simulink model "nav2"  (R2020a)
settings: Solver=FixedStepAuto  StartTime=0.0  StopTime=inf  RelTol=1e-3
model workspace (MAT data in the model file):
  SL_ROS_VariableLengthArrays_MaxSizes.CommonInfo.ArrayTruncateAction = 'EmitWarning'
  SL_ROS_VariableLengthArrays_MaxSizes.MsgTypeMap = containers.Map
  SL_ROS_VariableLengthArrays_MaxSizes.MsgTypeMap.serialization.keys = {'nav_msgs/OccupancyGrid'}
  SL_ROS_VariableLengthArrays_MaxSizes.MsgTypeMap.serialization.values{1}.PropertyName = 'Data'
  SL_ROS_VariableLengthArrays_MaxSizes.MsgTypeMap.serialization.values{1}.DataType = 'int8'
  SL_ROS_VariableLengthArrays_MaxSizes.MsgTypeMap.serialization.values{1}.MaxLength = 1000000
  SL_ROS_VariableLengthArrays_MaxSizes.MsgTypeMap.serialization.uniformity = 0
  SL_ROS_VariableLengthArrays_MaxSizes.MsgTypeMap.serialization.keyType = 'char'
  SL_ROS_VariableLengthArrays_MaxSizes.MsgTypeMap.serialization.valueType = 'any'
values from neighbouring files (symbols this model uses):
  chargingStn = [setInitialPose(1,1), setInitialPose(1,2)]    [startup.m]
  L2RTransform = [cos(L2Rtheta), -sin(L2Rtheta), L2Rx ... (first row only)    [startup.m]
  LIVE_MODE = 0    [startup.m]
  loadingStn = [15, 15]    [startup.m]
  map = binaryOccupancyMap(logicalMap, 1/0.05)    [exampleHelperVisualizeExecuteRobots.m]
  unloadingStn = [15, 15]    [startup.m]
  W2LOTransform = W2ORTransform/(L2RTransform)    [startup.m]
  wheelBase = 0.4464    [startup.m]
  wheelRadius = 0.1715/2    (= 0.08575)    [startup.m]
undefined symbols (not defined in the file or in its folder): Angular, gray, Linear
libraries: robotlib x7, robotalgslib x2, vrlib x1
settings Model: EnablePacing=on  Creator=john  LastModifiedBy=jhtran
settings OptimizationCC: EnhancedBackFolding=on  PassReuseOutputArgsAs=Individual arguments  ZeroExternalMemoryAtStartup=off  ZeroInternalMemoryAtStartup=off  MaxStackSize=64  OptimizeBlockOrder=speed  DifferentSizesBufferReuse=on  OptimizationCustomize=off  EfficientTunableParamExpr=on
settings DebuggingCC: ParameterTunabilityLossMsg=error
settings HardwareCC: ProdBitPerPointer=32  ProdBitPerSizeT=32  ProdBitPerPtrDiffT=32  ProdLargestAtomicFloat=None  ProdIntDivRoundTo=Undefined  ProdEndianess=Unspecified  ProdWordSize=32  ProdHWDeviceType=Generic->Unspecified (assume 32-bit Generic)  UseEmbeddedCoderFeatures=off
settings RTWCC: SystemTargetFile=ert.tlc  HardwareBoard=Robot Operating System (ROS)  TemplateMakefile=ert_default_tmf  Toolchain=Catkin  TargetLang=C++
settings CodeAppCC: ForceParamTrailComments=on  IgnoreCustomStorageClasses=off  OperatorAnnotations=on  SimulinkDataObjDesc=on  SFDataObjDesc=on  InsertBlockDesc=on
settings ERTTargetCC: SupportNonInlinedSFcns=on

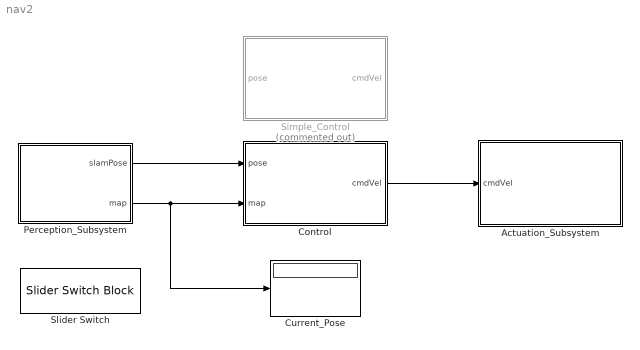
== system nav2 ==
  Actuation_Subsystem : Subsystem
  Control : Subsystem
  Current_Pose : Display
  Perception_Subsystem : Subsystem
  Simple_Control : Subsystem  Commented=on
  Slider Switch : SliderSwitchBlock
      settings: Values={{'Off', 'On'}, [0 1]}
  wires:
  Perception_Subsystem/1(slamPose) -> Control/1(pose)
  Control/1(cmdVel) -> Actuation_Subsystem/1(cmdVel)
  Perception_Subsystem/2(map) -> Current_Pose/1, Control/2(map)

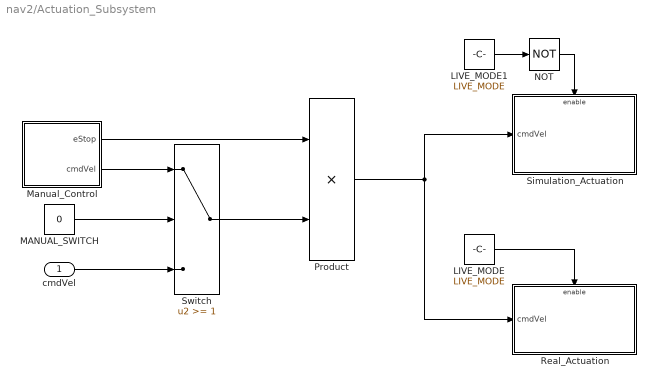
== system nav2/Actuation_Subsystem ==
  cmdVel : Inport
  LIVE_MODE : Constant  Value=LIVE_MODE
  LIVE_MODE1 : Constant  Value=LIVE_MODE
  MANUAL_SWITCH : Constant  Value=0
  Manual_Control : Subsystem
  NOT : Logic  Operator=NOT  IconShape=distinctive  AllPortsSameDT=off  OutDataTypeStr=boolean
  Product : Product
  Real_Actuation : Subsystem
  Simulation_Actuation : Subsystem
  Switch : Switch  Threshold=1
  wires:
  cmdVel/1 -> Switch/3
  Manual_Control/2(cmdVel) -> Switch/1
  MANUAL_SWITCH/1 -> Switch/2
  LIVE_MODE/1 -> Real_Actuation/Enable
  NOT/1 -> Simulation_Actuation/Enable
  LIVE_MODE1/1 -> NOT/1
  Switch/1 -> Product/2
  Product/1 -> Real_Actuation/1(cmdVel), Simulation_Actuation/1(cmdVel)
  Manual_Control/1(eStop) -> Product/1

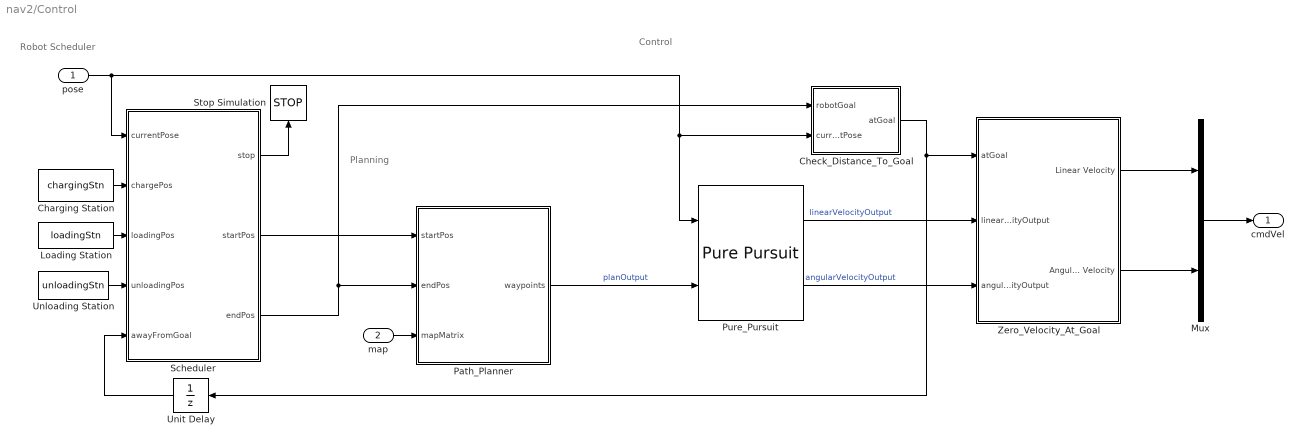
== system nav2/Control ==
  note: Control
  note: Robot Scheduler
  note: Planning
  pose : Inport
  map : Inport  Port=2
  "Charging Station " : Constant  Value=chargingStn  SampleTime=1
  Check_Distance_To_Goal : Subsystem
  Loading Station : Constant  Value=loadingStn
  Mux : Mux  Inputs=2
  Path_Planner : MATLAB Function  TreatAsAtomicUnit=on
  Pure_Pursuit : robotalgslib/Pure Pursuit  DesiredLinearVelocity=1  MaxAngularVelocity=0.5  LookaheadDistance=1  TargetDirPort=off  SimulateUsing=Code generation
  Scheduler : Stateflow chart  TreatAsAtomicUnit=on
  Stop Simulation : Stop
  Unit Delay : UnitDelay  SampleTime=-1  HasFrameUpgradeWarning=on
  Unloading Station : Constant  Value=unloadingStn  SampleTime=1
  Zero_Velocity_At_Goal : Subsystem
  cmdVel : Outport
  wires:
  Check_Distance_To_Goal/1(atGoal) -> Unit Delay/1, Zero_Velocity_At_Goal/1(atGoal)
  "Charging Station "/1 -> Scheduler/2(chargePos)
  Scheduler/2(startPos) -> Path_Planner/1(startPos)
  Unit Delay/1 -> Scheduler/5(awayFromGoal)
  Scheduler/3(endPos) -> Path_Planner/2(endPos), Check_Distance_To_Goal/1(robotGoal)
  Loading Station/1 -> Scheduler/3(loadingPos)
  Pure_Pursuit/2 -> Zero_Velocity_At_Goal/3(angularVelocityOutput)  "angularVelocityOutput"
  pose/1 -> Check_Distance_To_Goal/2(currentPose), Pure_Pursuit/1, Scheduler/1(currentPose)
  Unloading Station/1 -> Scheduler/4(unloadingPos)
  Scheduler/1(stop) -> Stop Simulation/1
  Path_Planner/1(waypoints) -> Pure_Pursuit/2  "planOutput"
  Pure_Pursuit/1 -> Zero_Velocity_At_Goal/2(linearVelocityOutput)  "linearVelocityOutput"
  Zero_Velocity_At_Goal/2(Angular Velocity) -> Mux/2
  Zero_Velocity_At_Goal/1(Linear Velocity) -> Mux/1
  Mux/1 -> cmdVel/1
  map/1 -> Path_Planner/3(mapMatrix)

== system nav2/Perception_Subsystem ==
  SLAM_Subsystem : Subsystem
  slamPose : Outport
  map : Outport  Port=2
  wires:
  SLAM_Subsystem/1(slamPose) -> slamPose/1
  SLAM_Subsystem/2(map) -> map/1

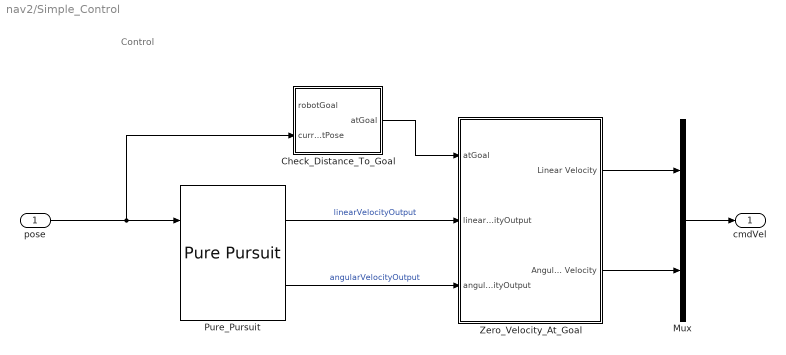
== system nav2/Simple_Control ==
  note: Control
  pose : Inport
  Check_Distance_To_Goal : Subsystem
  Mux : Mux  Inputs=2
  Pure_Pursuit : robotalgslib/Pure Pursuit  DesiredLinearVelocity=1  MaxAngularVelocity=0.5  LookaheadDistance=1  TargetDirPort=off  SimulateUsing=Code generation
  Zero_Velocity_At_Goal : Subsystem
  cmdVel : Outport
  wires:
  Check_Distance_To_Goal/1(atGoal) -> Zero_Velocity_At_Goal/1(atGoal)
  Pure_Pursuit/2 -> Zero_Velocity_At_Goal/3(angularVelocityOutput)  "angularVelocityOutput"
  Pure_Pursuit/1 -> Zero_Velocity_At_Goal/2(linearVelocityOutput)  "linearVelocityOutput"
  Zero_Velocity_At_Goal/2(Angular Velocity) -> Mux/2
  Zero_Velocity_At_Goal/1(Linear Velocity) -> Mux/1
  Mux/1 -> cmdVel/1
  pose/1 -> Check_Distance_To_Goal/2(currentPose), Pure_Pursuit/1
  ? -> Check_Distance_To_Goal/1(robotGoal)

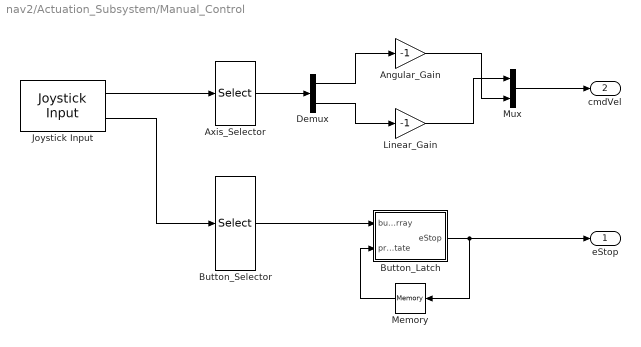
== system nav2/Actuation_Subsystem/Manual_Control ==
  Angular_Gain : Gain  Gain=-1
  Axis_Selector : Selector  InputPortWidth=8  IndexOptions=Index vector (dialog)  Indices=[1 2]  OutputSizes=1
  Button_Latch : MATLAB Function  TreatAsAtomicUnit=on
  Button_Selector : Selector  InputPortWidth=13  IndexOptions=Index vector (dialog)  Indices=[1 3]  OutputSizes=1
  Demux : Demux  Outputs=2
  Joystick Input : vrlib/Joystick Input  joyid=1  adjustports=on  forcefeed=off
  Linear_Gain : Gain  Gain=-1
  Memory : Memory  InitialCondition=1
  Mux : Mux  Inputs=2
  eStop : Outport
  cmdVel : Outport  Port=2
  wires:
  Demux/1 -> Angular_Gain/1
  Axis_Selector/1 -> Demux/1
  Demux/2 -> Linear_Gain/1
  Joystick Input/1 -> Axis_Selector/1
  Linear_Gain/1 -> Mux/1
  Angular_Gain/1 -> Mux/2
  Mux/1 -> cmdVel/1
  Joystick Input/2 -> Button_Selector/1
  Memory/1 -> Button_Latch/2(prevEState)
  Button_Selector/1 -> Button_Latch/1(buttonArray)
  Button_Latch/1(eStop) -> eStop/1, Memory/1

== system nav2/Actuation_Subsystem/Real_Actuation ==
  cmdVel : Inport
  Enable : EnablePort
  Actuator : Subsystem
  Demux : Demux  Outputs=2
  Forward Kinematics : Subsystem
  wires:
  Forward Kinematics/1(leftRpmOut) -> Actuator/1(leftRPM)
  Demux/1 -> Forward Kinematics/1(v_in)
  Forward Kinematics/2(rightRpmOut) -> Actuator/2(rightRPM)
  Demux/2 -> Forward Kinematics/2(w_in)
  cmdVel/1 -> Demux/1

== system nav2/Actuation_Subsystem/Simulation_Actuation ==
  cmdVel : Inport
  Enable : EnablePort
  Blank Message : robotlib/Blank Message  messageClass=Message  entityType=geometry_msgs/Twist  messageType=geometry_msgs/Twist  SampleTime=inf
  Bus Assignment : BusAssignment  AssignedSignals=Linear.X,Angular.Z
  Demux : Demux  Outputs=2
  Publish : robotlib/Publish  topicSource=Select from ROS network  topic=/sim_cmd_vel  messageType=geometry_msgs/Twist  messageQueueLength=1
  wires:
  Blank Message/1 -> Bus Assignment/1
  Bus Assignment/1 -> Publish/1
  Demux/2 -> Bus Assignment/3
  Demux/1 -> Bus Assignment/2
  cmdVel/1 -> Demux/1

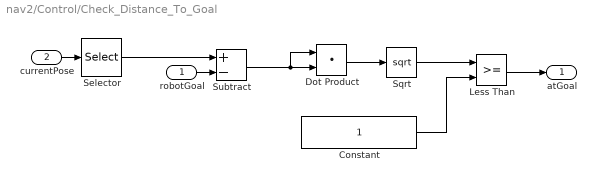
== system nav2/Control/Check_Distance_To_Goal ==
  robotGoal : Inport
  currentPose : Inport  Port=2
  Constant : Constant
  Dot Product : DotProduct  InputSameDT=on  OutDataTypeStr=Inherit: Inherit via internal rule
  Less Than : RelationalOperator  OutDataTypeStr=boolean  RndMeth=Simplest
  Selector : Selector  InputPortWidth=3  IndexOptions=Index vector (dialog)  Indices=[1 2]  OutputSizes=1
  Sqrt : Sqrt  SaturateOnIntegerOverflow=on
  Subtract : Sum  Inputs=+-
  atGoal : Outport
  wires:
  robotGoal/1 -> Subtract/2
  Dot Product/1 -> Sqrt/1
  Constant/1 -> Less Than/2
  currentPose/1 -> Selector/1
  Less Than/1 -> atGoal/1
  Sqrt/1 -> Less Than/1
  Subtract/1 -> Dot Product/1, Dot Product/2
  Selector/1 -> Subtract/1

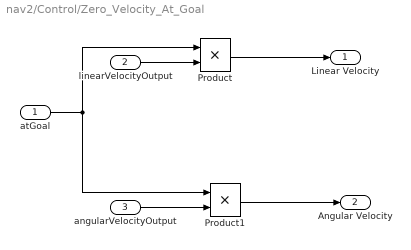
== system nav2/Control/Zero_Velocity_At_Goal ==
  atGoal : Inport
  linearVelocityOutput : Inport  Port=2
  angularVelocityOutput : Inport  Port=3
  Product : Product
  Product1 : Product
  Linear Velocity : Outport  OutDataTypeStr=double
  Angular Velocity : Outport  Port=2  OutDataTypeStr=double
  wires:
  atGoal/1 -> Product1/1, Product/1
  angularVelocityOutput/1 -> Product1/2
  linearVelocityOutput/1 -> Product/2
  Product/1 -> Linear Velocity/1
  Product1/1 -> Angular Velocity/1

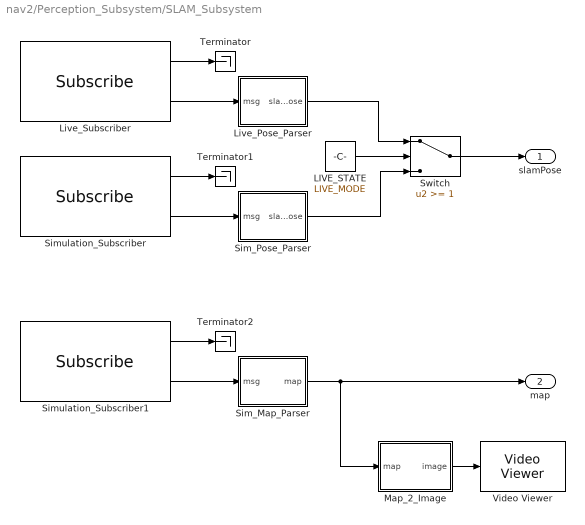
== system nav2/Perception_Subsystem/SLAM_Subsystem ==
  LIVE_STATE : Constant  Value=LIVE_MODE
  Live_Pose_Parser : Subsystem
  Live_Subscriber : robotlib/Subscribe  topicSource=Select from ROS network  topic=/slamware_ros_sdk_server_node/odom  messageType=nav_msgs/Odometry  sampleTime=-1  messageQueueLength=1
  Map_2_Image : MATLAB Function  TreatAsAtomicUnit=on
  Sim_Map_Parser : Subsystem
  Sim_Pose_Parser : Subsystem
  Simulation_Subscriber : robotlib/Subscribe  topicSource=Select from ROS network  topic=/odom  messageType=nav_msgs/Odometry  sampleTime=-1  messageQueueLength=1
  Simulation_Subscriber1 : robotlib/Subscribe  topicSource=Select from ROS network  topic=/map  messageType=nav_msgs/OccupancyGrid  sampleTime=-1  messageQueueLength=1
  Switch : Switch  Threshold=1
  Terminator : Terminator
  Terminator1 : Terminator
  Terminator2 : Terminator
  Video Viewer : VideoViewer  colormapValue=gray(256)  FigPos=[1104 867 693 501]
  slamPose : Outport
  map : Outport  Port=2
  wires:
  LIVE_STATE/1 -> Switch/2
  Live_Subscriber/2 -> Live_Pose_Parser/1(msg)
  Simulation_Subscriber/2 -> Sim_Pose_Parser/1(msg)
  Sim_Pose_Parser/1(slamPose) -> Switch/3
  Live_Pose_Parser/1(slamPose) -> Switch/1
  Switch/1 -> slamPose/1
  Simulation_Subscriber/1 -> Terminator1/1
  Live_Subscriber/1 -> Terminator/1
  Simulation_Subscriber1/2 -> Sim_Map_Parser/1(msg)
  Sim_Map_Parser/1(map) -> map/1, Map_2_Image/1(map)
  Map_2_Image/1(image) -> Video Viewer/1
  Simulation_Subscriber1/1 -> Terminator2/1

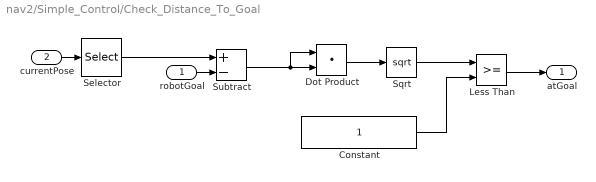
== system nav2/Simple_Control/Check_Distance_To_Goal ==
  robotGoal : Inport
  currentPose : Inport  Port=2
  Constant : Constant
  Dot Product : DotProduct  InputSameDT=on  OutDataTypeStr=Inherit: Inherit via internal rule
  Less Than : RelationalOperator  OutDataTypeStr=boolean  RndMeth=Simplest
  Selector : Selector  InputPortWidth=3  IndexOptions=Index vector (dialog)  Indices=[1 2]  OutputSizes=1
  Sqrt : Sqrt  SaturateOnIntegerOverflow=on
  Subtract : Sum  Inputs=+-
  atGoal : Outport
  wires:
  robotGoal/1 -> Subtract/2
  Dot Product/1 -> Sqrt/1
  Constant/1 -> Less Than/2
  currentPose/1 -> Selector/1
  Less Than/1 -> atGoal/1
  Sqrt/1 -> Less Than/1
  Subtract/1 -> Dot Product/1, Dot Product/2
  Selector/1 -> Subtract/1

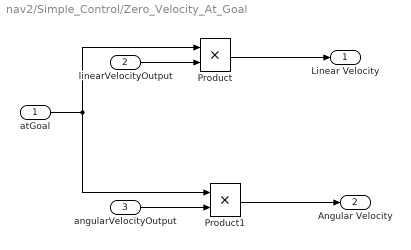
== system nav2/Simple_Control/Zero_Velocity_At_Goal ==
  atGoal : Inport
  linearVelocityOutput : Inport  Port=2
  angularVelocityOutput : Inport  Port=3
  Product : Product
  Product1 : Product
  Linear Velocity : Outport  OutDataTypeStr=double
  Angular Velocity : Outport  Port=2  OutDataTypeStr=double
  wires:
  atGoal/1 -> Product1/1, Product/1
  angularVelocityOutput/1 -> Product1/2
  linearVelocityOutput/1 -> Product/2
  Product/1 -> Linear Velocity/1
  Product1/1 -> Angular Velocity/1

== system nav2/Actuation_Subsystem/Real_Actuation/Actuator ==
  leftRPM : Inport
  rightRPM : Inport  Port=2
  Blank Message : robotlib/Blank Message  messageClass=Message  entityType=geometry_msgs/Twist  messageType=geometry_msgs/Twist  SampleTime=inf
  Bus Assignment : BusAssignment  AssignedSignals=Angular.X,Angular.Y
  Publish : robotlib/Publish  topicSource=Select from ROS network  topic=/zlac8015d/rpm  messageType=geometry_msgs/Twist  messageQueueLength=1
  wires:
  Bus Assignment/1 -> Publish/1
  Blank Message/1 -> Bus Assignment/1
  rightRPM/1 -> Bus Assignment/3
  leftRPM/1 -> Bus Assignment/2

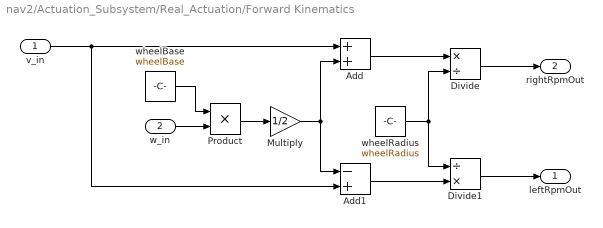
== system nav2/Actuation_Subsystem/Real_Actuation/Forward Kinematics ==
  v_in : Inport
  w_in : Inport  Port=2
  Add : Sum
  Add1 : Sum  Inputs=-+
  Divide : Product  Inputs=*/
  Divide1 : Product  Inputs=/*
  Multiply : Gain  Gain=1/2
  Product : Product
  wheelBase : Constant  Value=wheelBase
  wheelRadius : Constant  Value=wheelRadius
  leftRpmOut : Outport
  rightRpmOut : Outport  Port=2
  wires:
  v_in/1 -> Add1/2, Add/1
  w_in/1 -> Product/2
  wheelBase/1 -> Product/1
  Product/1 -> Multiply/1
  Multiply/1 -> Add/2, Add1/1
  Add1/1 -> Divide1/2
  Add/1 -> Divide/1
  wheelRadius/1 -> Divide1/1, Divide/2
  Divide1/1 -> leftRpmOut/1
  Divide/1 -> rightRpmOut/1

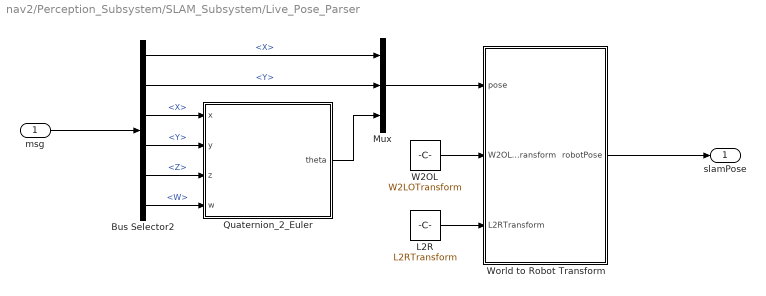
== system nav2/Perception_Subsystem/SLAM_Subsystem/Live_Pose_Parser ==
  msg : Inport
  Bus Selector2 : BusSelector  OutputSignals=Pose.Pose.Position.X,Pose.Pose.Position.Y,Pose.Pose.Orientation.X,Pose.Pose.Orientation.Y,Pose.Pose.Orientation.Z,Pose.Pose.Orientation.W
  L2R : Constant  Value=L2RTransform
  Mux : Mux  Inputs=3
  Quaternion_2_Euler : MATLAB Function  TreatAsAtomicUnit=on
  W2OL : Constant  Value=W2LOTransform
  World to Robot Transform : MATLAB Function  TreatAsAtomicUnit=on
  slamPose : Outport
  wires:
  msg/1 -> Bus Selector2/1
  Bus Selector2/1 -> Mux/1  "<X>"
  Bus Selector2/2 -> Mux/2  "<Y>"
  Bus Selector2/3 -> Quaternion_2_Euler/1(x)  "<X>"
  Bus Selector2/4 -> Quaternion_2_Euler/2(y)  "<Y>"
  Bus Selector2/5 -> Quaternion_2_Euler/3(z)  "<Z>"
  Bus Selector2/6 -> Quaternion_2_Euler/4(w)  "<W>"
  Quaternion_2_Euler/1(theta) -> Mux/3
  Mux/1 -> World to Robot Transform/1(pose)
  World to Robot Transform/1(robotPose) -> slamPose/1
  W2OL/1 -> World to Robot Transform/2(W2OLTransform)
  L2R/1 -> World to Robot Transform/3(L2RTransform)

== system nav2/Perception_Subsystem/SLAM_Subsystem/Sim_Map_Parser ==
  msg : Inport
  Bus Selector2 : BusSelector  OutputSignals=Data,Info.Width,Info.Height
  Map_Parser : MATLAB Function  TreatAsAtomicUnit=on
  map : Outport
  wires:
  msg/1 -> Bus Selector2/1
  Bus Selector2/1 -> Map_Parser/1(mapArray)  "<Data>"
  Map_Parser/1(logicalMatrix) -> map/1
  Bus Selector2/2 -> Map_Parser/2(mapWidth)  "<Width>"
  Bus Selector2/3 -> Map_Parser/3(mapHeight)  "<Height>"

== system nav2/Perception_Subsystem/SLAM_Subsystem/Sim_Pose_Parser ==
  msg : Inport
  Bus Selector2 : BusSelector  OutputSignals=Pose.Pose.Position.X,Pose.Pose.Position.Y,Pose.Pose.Orientation.X,Pose.Pose.Orientation.Y,Pose.Pose.Orientation.Z,Pose.Pose.Orientation.W
  Mux : Mux  Inputs=3
  Quaternion_2_Euler : MATLAB Function  TreatAsAtomicUnit=on
  slamPose : Outport
  wires:
  msg/1 -> Bus Selector2/1
  Mux/1 -> slamPose/1
  Bus Selector2/1 -> Mux/1  "<X>"
  Bus Selector2/2 -> Mux/2  "<Y>"
  Bus Selector2/3 -> Quaternion_2_Euler/1(x)  "<X>"
  Bus Selector2/4 -> Quaternion_2_Euler/2(y)  "<Y>"
  Bus Selector2/5 -> Quaternion_2_Euler/3(z)  "<Z>"
  Bus Selector2/6 -> Quaternion_2_Euler/4(w)  "<W>"
  Quaternion_2_Euler/1(theta) -> Mux/3

== matlab function nav2/Perception_Subsystem/SLAM_Subsystem/Sim_Pose_Parser/Quaternion_2_Euler ==
  data: x input; theta output; y input; z input; w input
function theta = fcn(x, y, z, w)

    euler = quat2eul([x, y, z, w]); 
    
    if sum(isnan(euler)) == 3
        
        euler = ([pi, 0, 0]);
        
    end 
    
theta = euler(1,3);

== matlab function nav2/Perception_Subsystem/SLAM_Subsystem/Sim_Map_Parser/Map_Parser ==
  data: mapArray input; logicalMatrix output size=[1000,1000]; mapWidth input; mapHeight input
function logicalMatrix = fcn(mapArray, mapWidth, mapHeight)

index = 1; 

% Check if width is larger then height
if mapWidth < mapHeight
    mapMatrix = zeros(mapHeight, 'int8'); 
else
    mapMatrix = zeros(mapWidth, 'int8'); 
end

% Remap 
for i = 1:mapHeight
    for j = 1:mapWidth 
        mapMatrix(i,j) = mapArray(index);
        index = index + 1; 
    end
end


logicalMatrix = imcomplement(mapMatrix < 100);

== matlab function nav2/Control/Path_Planner ==
  settings: updateMethod=DISCRETE
  data: startPos input size=[1 2]; endPos input size=[1 2]; waypoints output size=[500 2]; mapMatrix input
function waypoints = planning(startPos, endPos, mapMatrix)

persistent waypointsInternal
persistent prevStartPos
persistent prevEndPos

% Set constant parameters
maxNumNodes = 500;
robotLength = 0.775;

% Initialize persistent variables that are used downstream
if isempty(prevStartPos)
    prevStartPos = startPos;
end

if isempty(prevEndPos)
    prevEndPos = endPos;
end

isNewPath = (~isequal(prevStartPos, startPos) || ~isequal(prevEndPos, endPos));

if isempty(waypointsInternal) || isNewPath
    % Two conditions in which waypoints must be set: they are not yet
    % initialized, or they are initialized, but the current start and end
    % do not match those used to generate the previous set of waypoints
    [waypointsInternal] = planPath(mapMatrix, maxNumNodes, startPos, endPos);
end

% Update the outputs
waypoints = waypointsInternal;

% Update the persistent variables that indicate previous state
prevStartPos = startPos;
prevEndPos = endPos;

%% Helper Function

function wayPoints = planPath(mapMatrix, maxNodes, startPos, endPos)
    
    % Create a probabilistic roadmap
    map = binaryOccupancyMap(mapMatrix, 1/0.05);
    inflate(map, robotLength/2);
    prm = mobileRobotPRM(map, maxNodes);
    
    % Find a path between two points
    xy = findpath(prm, startPos(:)', endPos(:)');
    wayPoints = repmat(endPos(:)', maxNodes, 1);
    
    % Number of nodes that are actually used
    numNodes = length(xy);
    wayPoints(1:numNodes,:) = xy;    

end

end

== matlab function nav2/Perception_Subsystem/SLAM_Subsystem/Live_Pose_Parser/World to Robot Transform ==
  data: pose input; robotPose output; W2OLTransform input; L2RTransform input
function robotPose = fcn(pose, W2OLTransform, L2RTransform)
    
    % O2L Transform 
    OL2LTransform = [cos(pose(3,1)), -sin(pose(3,1)), pose(1,1);
                    sin(pose(3,1)), cos(pose(3,1)), pose(2,1);
                    0,              0,              1];

    % Calculate World to Robot
    W2RTransform = W2OLTransform*OL2LTransform*L2RTransform; 
    

    % Extract relevant information
robotPose = [W2RTransform(1,3); W2RTransform(2,3); acos(W2RTransform(1,1))];

== matlab function nav2/Perception_Subsystem/SLAM_Subsystem/Map_2_Image ==
  data: map input; image output size=[1000,1000]
function image = fcn(map)

image = imcomplement(flipud(map));

== matlab function nav2/Actuation_Subsystem/Manual_Control/Button_Latch ==
  data: buttonArray input; prevEState input; eStop output
function eStop = fcn(buttonArray, prevEState)

    % Copy previous E State
    currentEState = prevEState; 

    % Map Button Array
    eStopButton = buttonArray(1,1); 
    resetStopButton = buttonArray(2,1); 

    % Check if emergency button is pressed and st
    if eStopButton == 1
        
        % Set stop state to be 0
        currentEState = 0;
        
    % Check if reset button is pressed
    elseif resetStopButton == 1
        
        % Set stop state to be 0 
        currentEState = 1; 
        
    end

eStop = currentEState;

== matlab function nav2/Perception_Subsystem/SLAM_Subsystem/Live_Pose_Parser/Quaternion_2_Euler ==
  data: x input; theta output; y input; z input; w input
function theta = fcn(x, y, z, w)

    euler = quat2eul([x, y, z, w]); 
    
    if sum(isnan(euler)) == 3
        
        euler = ([pi, 0, 0]);
        
    end 
    
theta = euler(1,3);

== stateflow chart nav2/Control/Scheduler ==
  settings: sampleTime=0.01
  state Unloading
    entry, during:
    endPos = unloadingPos';
  state Loading
    entry,during:
    endPos = loadingPos';
  state Charging
    entry, during:
    endPos = chargePos';
  (default) -> Loading : {startPos = chargePos';}
  Loading -> Unloading : [~awayFromGoal && after(stopDelay, tick)]
      |
      | {startPos = currentPose(1:2)';}
  Unloading -> Charging : [~awayFromGoal  && after(stopDelay, tick)]
      | {startPos = currentPose(1:2)';}
  Charging -> (junction 201) : [~awayFromGoal]{stop = 1;}
  data: currentPose input; stop output =0; chargePos input size=[2 1]; loadingPos input size=[2 1]; unloadingPos input size=[2 1]; startPos output size=[1, 2]; endPos output size=[1, 2]; awayFromGoal input; stopDelay local =5
